simulink model "My_System"  (R2022b)
settings: Solver=ode4  StartTime=0.0  StopTime=10.0  FixedStep=0.01  RelTol=1e-3  EnableMultiTasking=on
Description:
  | Real-Time Van der Pol Simulation
  | 
  | This demonstration shows a real-time version of the Simulink Van der Pol
  | simulation demo. This model does not need any external signals, so it does
  | not need any data acquisition hardware or driver. This makes the model ideal
  | for first experiments with Real-Time Windows Target, without need to
  | worry about proper I/O hardware configuration.
  | 
  | How to run this demo:
  | 
  |   1. Build the model using Tools -> Real-Time Workshop -> Build Model.
  |   2. Connect to the real-time code using Simulation -> Connect to target.
  |   3. Start the real-time execution using Simulation -> Start real-time code.
settings Model: SimulationMode=external  Creator=Houska  LastModifiedBy=artur
settings SolverCC: AlgebraicLoopSolver=TrustRegion
settings DataIOCC: LimitDataPoints=on  SaveFormat=Array  SignalLoggingSaveFormat=ModelDataLogs  SaveOutput=off  SaveTime=off  ReturnWorkspaceOutputs=off  SignalLoggingName=logsOut
settings OptimizationCC: ExpressionDepthLimit=2147483647  InitFltsAndDblsToZero=on
settings DebuggingCC: SaveWithParameterizedLinksMsg=none  UnderspecifiedInitializationDetection=Classic  MergeDetectMultiDrivingBlocksExec=none  SignalResolutionControl=TryResolveAllWithWarning  MultiTaskDSMMsg=warning  MultiTaskCondExecSysMsg=none  FcnCallInpInsideContextMsg=warning  UnconnectedInputMsg=warning  UnconnectedOutputMsg=warning  UnconnectedLineMsg=warning  AllowSymbolicDim=off  StateNameClashWarn=warning  PregeneratedLibrarySubsystemCodeDiagnostic=none  SFUnexpectedBacktrackingDiag=warning  SFNoUnconditionalDefaultTransitionDiag=warning  SFExecutionAtInitializationDiag=none  SFMachineParentedDataDiag=warning  ArithmeticOperatorsInVariantConditions=warning
settings HardwareCC: ProdBitPerPointer=32  ProdBitPerSizeT=32  ProdBitPerPtrDiffT=32  ProdLargestAtomicFloat=None  ProdWordSize=32  ProdHWDeviceType=32-bit Real-Time Windows Target  TargetHWDeviceType=32-bit Generic  ProdEqTarget=off
settings ModelReferenceCC: EnableRefExpFcnMdlSchedulingChecks=on  PropagateSignalLabelsOutOfModel=off
settings SFSimCC: SimUseLocalCustomCode=off  CustomCodeUndefinedFunction=UseInterfaceOnly
settings RTWCC: Description=servo (Visual C/C++)  SystemTargetFile=rtcon_servo_usb2.tlc  TemplateMakefile=servo_vc_usb2_x64.tmf  RTWUseLocalCustomCode=off  DLArmComputeVersion=19.05
settings CodeAppCC: StateflowObjectComments=on
settings STFCustomTargetCC: ModelReferenceCompliant=off  CombineOutputUpdateFcns=on  MatFileLogging=on  SystemTargetFile=rtcon_servo_usb2.tlc
settings GRTTargetCC: TargetLangStandard=C89/C90 (ANSI)  ModelReferenceCompliant=off  ParMdlRefBuildCompliant=off  CompOptLevelCompliant=off  ConcurrentExecutionCompliant=off  CPPClassGenCompliant=off  UseToolchainInfoCompliant=off  ExtMode=on  ExtModeMexFile=rtcon_ext_comm
settings ConfigComp: CovMetricSettings=dw  CovSaveCumulativeToWorkspaceVar=on  CovSaveSingleToWorkspaceVar=on  CovExternalEMLEnable=off  CovSFcnEnable=off

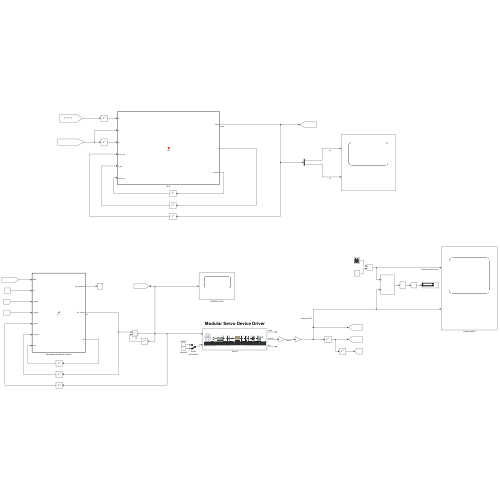
[thumbnail: Simulink's stored preview of the top-level diagram]
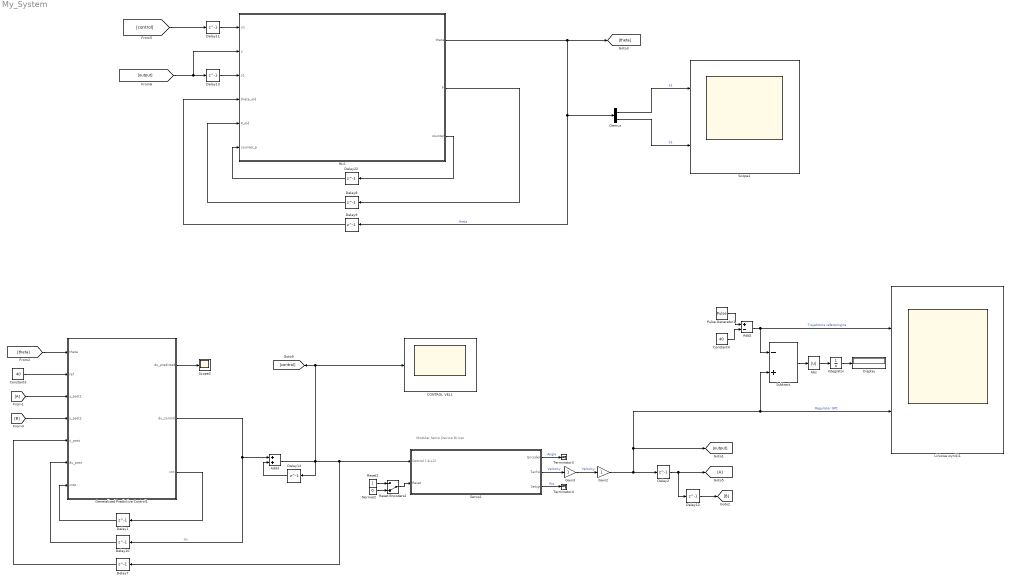
== system My_System ==
  note: Modular Servo Device Driver
  Abs : Abs  SaturateOnIntegerOverflow=off
  Add2 : Sum  Inputs=+-
  Add3 : Sum
  CONTROL VEL1 : Scope
  Constant3 : Constant  Value=40
  Constant4 : Constant  Value=40
  Delay1 : Delay  DelayLength=1  InitialCondition=1
  Delay{2,7,10..14} (7 alike) : Delay  DelayLength=1  InitialCondition=0
  Delay22 : Delay  DelayLength=1  InitialCondition=10
  Delay8 : Delay  DelayLength=1  InitialCondition=eye(2) * 10^6
  Delay9 : Delay  DelayLength=1  InitialCondition=[0.79 1.9048]
  Demux : Demux  Outputs=2
  Display : Display
  From1 : From
  Gain2 : Gain
  Gain3 : Gain
  Generalized Predictive Control1 : MATLAB Function  TreatAsAtomicUnit=on
  Goto5 : Goto
  Integrator : Integrator
  Liniowe wyniki1 : Scope  NumInputPorts=2
  Normal2 : Constant  Value=0
  Pulse Generator1 : DiscretePulseGenerator  PulseType=Time based  Amplitude=80  Period=4  PulseWidth=50
  RLS : MATLAB Function  TreatAsAtomicUnit=on
  Reset Encoders2 : ManualSwitch  CurrentSetting=0
  Reset2 : Constant
  Scope1 : Scope  NumInputPorts=2
  Scope2 : Scope
  Servo2 : Subsystem
      mask Display: image(imread('Servo_inteco.JPG'))
  Subtract : Sum  Inputs=-+
  Terminator3 : Terminator
  Terminator4 : Terminator
  wires:
  [control] -> Delay11/1
  RLS/1(theta) -> Demux/1, Delay9/1, [theta]  "theta"
  Delay9/1 -> RLS/4(theta_old)
  Delay8/1 -> RLS/5(P_old)
  [output] -> Delay13/1, RLS/2(y)
  Demux/2 -> Scope1/2  "b1"
  Delay13/1 -> RLS/3(y1)
  Delay22/1 -> RLS/6(counter_p)
  RLS/3(counter) -> Delay22/1
  Delay11/1 -> RLS/1(u1)
  Demux/1 -> Scope1/1  "a1"
  RLS/2(P) -> Delay8/1
  Generalized Predictive Control1/1(du_predicted) -> Scope2/1
  [B] -> Generalized Predictive Control1/4(y_past2)
  From1/1 -> Generalized Predictive Control1/3(y_past1)
  Generalized Predictive Control1/3(cnt) -> Delay1/1
  Gain2/1 -> Delay2/1, [output], Liniowe wyniki1/2, Subtract/2  "Regulator GPC"
  Constant4/1 -> Add2/2
  Delay12/1 -> [B]
  Delay2/1 -> Delay12/1, Goto5/1
  Subtract/1 -> Abs/1
  Delay10/1 -> Generalized Predictive Control1/6(du_past)
  Delay14/1 -> Add3/2
  [theta] -> Generalized Predictive Control1/1(theta)
  Generalized Predictive Control1/2(du_control) -> Delay10/1, Add3/1  "du"
  Add2/1 -> Liniowe wyniki1/1, Subtract/1  "Trajektoria referencyjna"
  Delay7/1 -> Generalized Predictive Control1/5(u_past)
  Delay1/1 -> Generalized Predictive Control1/7(cntp)
  Abs/1 -> Integrator/1
  Constant3/1 -> Generalized Predictive Control1/2(ref)
  Gain3/1 -> Gain2/1  "Velocity"
  Pulse Generator1/1 -> Add2/1
  Integrator/1 -> Display/1
  Servo2/2(Tacho) -> Gain3/1  "Velocity"
  Servo2/3(Setup) -> Terminator4/1  "Pot"
  Add3/1 -> [control], CONTROL VEL1/1, Servo2/1(Control (-1/+1)), Delay7/1, Delay14/1
  Reset Encoders2/1 -> Servo2/2(Reset)
  Servo2/1(Encoder) -> Terminator3/1  "Angle"
  Normal2/1 -> Reset Encoders2/2
  Reset2/1 -> Reset Encoders2/1

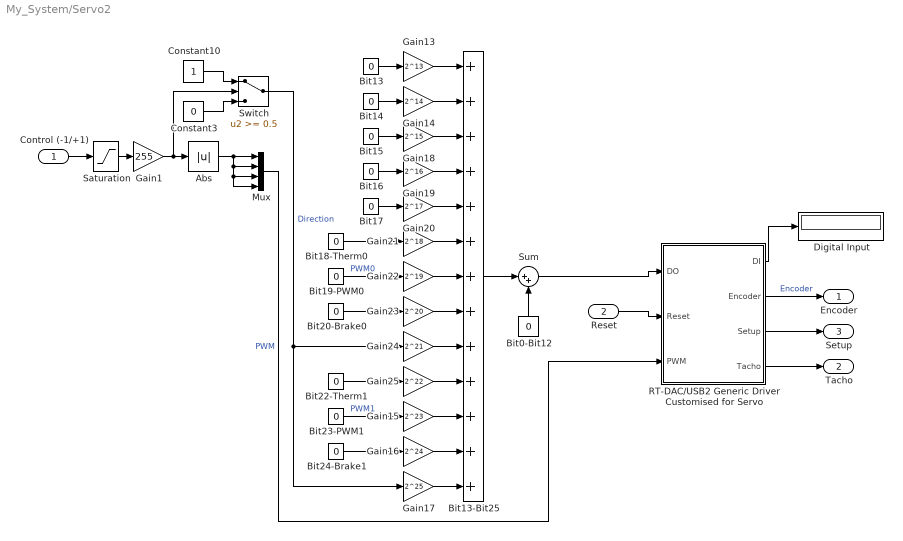
== system My_System/Servo2 ==
  Control (-1/+1) : Inport
  Reset : Inport  Port=2
  Abs : Abs
  Bit0-Bit12 : Constant  Value=0
  Bit{13..17} (5 alike) : Constant  Value=0
  Bit13-Bit25 : Sum  Inputs=+++++++++++++  InputSameDT=on  SaturateOnIntegerOverflow=on  OutDataTypeStr=Inherit: Same as first input
  Bit18-Therm0 : Constant  Value=0
  Bit19-PWM0 : Constant  Value=0
  Bit20-Brake0 : Constant  Value=0
  Bit22-Therm1 : Constant  Value=0
  Bit23-PWM1 : Constant  Value=0
  Bit24-Brake1 : Constant  Value=0
  Constant10 : Constant
  Constant3 : Constant  Value=0
  Digital Input : Display
  Gain1 : Gain  Gain=255  SaturateOnIntegerOverflow=on  OutDataTypeStr=Inherit: Same as input  ParamDataTypeStr=Inherit: Same as input
  Gain13 : Gain  Gain=2^13  SaturateOnIntegerOverflow=on  OutDataTypeStr=Inherit: Same as input  ParamDataTypeStr=Inherit: Same as input
  Gain14 : Gain  Gain=2^14  SaturateOnIntegerOverflow=on  OutDataTypeStr=Inherit: Same as input  ParamDataTypeStr=Inherit: Same as input
  Gain15 : Gain  Gain=2^23  SaturateOnIntegerOverflow=on  OutDataTypeStr=Inherit: Same as input  ParamDataTypeStr=Inherit: Same as input
  Gain16 : Gain  Gain=2^24  SaturateOnIntegerOverflow=on  OutDataTypeStr=Inherit: Same as input  ParamDataTypeStr=Inherit: Same as input
  Gain17 : Gain  Gain=2^25  SaturateOnIntegerOverflow=on  OutDataTypeStr=Inherit: Same as input  ParamDataTypeStr=Inherit: Same as input
  Gain18 : Gain  Gain=2^15  SaturateOnIntegerOverflow=on  OutDataTypeStr=Inherit: Same as input  ParamDataTypeStr=Inherit: Same as input
  Gain19 : Gain  Gain=2^16  SaturateOnIntegerOverflow=on  OutDataTypeStr=Inherit: Same as input  ParamDataTypeStr=Inherit: Same as input
  Gain20 : Gain  Gain=2^17  SaturateOnIntegerOverflow=on  OutDataTypeStr=Inherit: Same as input  ParamDataTypeStr=Inherit: Same as input
  Gain21 : Gain  Gain=2^18  SaturateOnIntegerOverflow=on  OutDataTypeStr=Inherit: Same as input  ParamDataTypeStr=Inherit: Same as input
  Gain22 : Gain  Gain=2^19  SaturateOnIntegerOverflow=on  OutDataTypeStr=Inherit: Same as input  ParamDataTypeStr=Inherit: Same as input
  Gain23 : Gain  Gain=2^20  SaturateOnIntegerOverflow=on  OutDataTypeStr=Inherit: Same as input  ParamDataTypeStr=Inherit: Same as input
  Gain24 : Gain  Gain=2^21  SaturateOnIntegerOverflow=on  OutDataTypeStr=Inherit: Same as input  ParamDataTypeStr=Inherit: Same as input
  Gain25 : Gain  Gain=2^22  SaturateOnIntegerOverflow=on  OutDataTypeStr=Inherit: Same as input  ParamDataTypeStr=Inherit: Same as input
  Mux : Mux
  RT-DAC/USB2 Generic Driver Customised for Servo : Subsystem
      mask Display: disp('RT-DAC/USB2\n\nGeneric Driver\nVersion 2.1')
  Saturation : Saturate  UpperLimit=1  LowerLimit=-1
  Sum : Sum  Inputs=|++  InputSameDT=on  SaturateOnIntegerOverflow=on  OutDataTypeStr=Inherit: Same as first input
  Switch : Switch  Threshold=0.5  SaturateOnIntegerOverflow=off
  Encoder : Outport  VectorParamsAs1DForOutWhenUnconnected=off
  Tacho : Outport  Port=2  VectorParamsAs1DForOutWhenUnconnected=off
  Setup : Outport  Port=3  VectorParamsAs1DForOutWhenUnconnected=off
  wires:
  RT-DAC/USB2 Generic Driver Customised for Servo/4(Tacho) -> Tacho/1
  RT-DAC/USB2 Generic Driver Customised for Servo/3(Setup) -> Setup/1
  RT-DAC/USB2 Generic Driver Customised for Servo/2(Encoder) -> Encoder/1  "Encoder"
  Mux/1 -> RT-DAC/USB2 Generic Driver Customised for Servo/3(PWM)  "PWM"
  Switch/1 -> Gain17/1, Gain24/1  "Direction"
  Abs/1 -> Mux/4, Mux/3, Mux/2, Mux/1
  Constant3/1 -> Switch/3
  Constant10/1 -> Switch/1
  Gain1/1 -> Switch/2, Abs/1
  Saturation/1 -> Gain1/1
  Control (-1/+1)/1 -> Saturation/1
  Reset/1 -> RT-DAC/USB2 Generic Driver Customised for Servo/2(Reset)
  Bit24-Brake1/1 -> Gain16/1
  Bit23-PWM1/1 -> Gain15/1  "PWM1"
  Bit22-Therm1/1 -> Gain25/1
  Bit13-Bit25/1 -> Sum/1
  Sum/1 -> RT-DAC/USB2 Generic Driver Customised for Servo/1(DO)
  Gain17/1 -> Bit13-Bit25/13
  Gain16/1 -> Bit13-Bit25/12
  Gain15/1 -> Bit13-Bit25/11
  Gain25/1 -> Bit13-Bit25/10
  Gain24/1 -> Bit13-Bit25/9
  Gain23/1 -> Bit13-Bit25/8
  Gain22/1 -> Bit13-Bit25/7
  Gain21/1 -> Bit13-Bit25/6
  Gain20/1 -> Bit13-Bit25/5
  Gain19/1 -> Bit13-Bit25/4
  Gain18/1 -> Bit13-Bit25/3
  Gain14/1 -> Bit13-Bit25/2
  Gain13/1 -> Bit13-Bit25/1
  Bit0-Bit12/1 -> Sum/2
  RT-DAC/USB2 Generic Driver Customised for Servo/1(DI) -> Digital Input/1
  Bit20-Brake0/1 -> Gain23/1
  Bit19-PWM0/1 -> Gain22/1  "PWM0"
  Bit18-Therm0/1 -> Gain21/1
  Bit17/1 -> Gain20/1
  Bit16/1 -> Gain19/1
  Bit15/1 -> Gain18/1
  Bit14/1 -> Gain14/1
  Bit13/1 -> Gain13/1

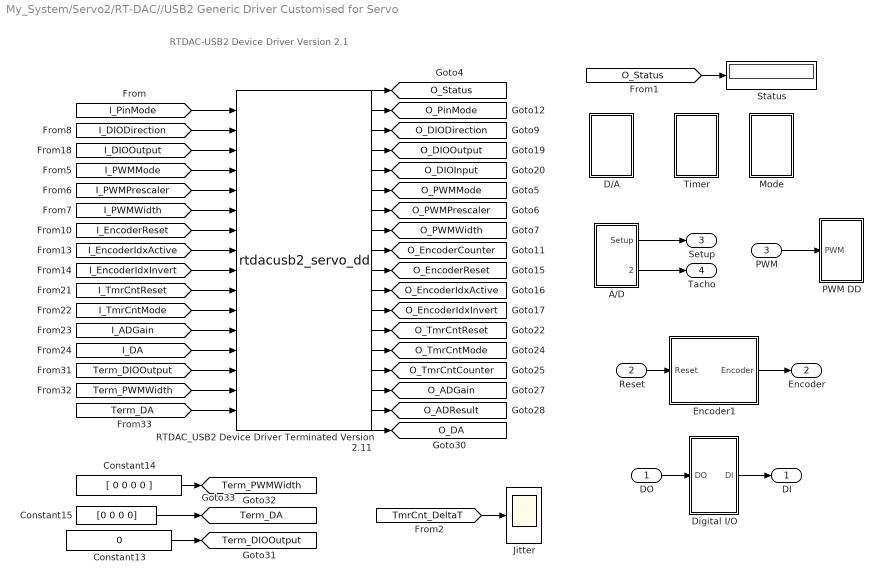
== system My_System/Servo2/RT-DAC//USB2 Generic Driver Customised for Servo ==
  note: RTDAC-USB2 Device Driver
      | Version 2.1
  DO : Inport
  Reset : Inport  Port=2
  PWM : Inport  Port=3
  A/D : Subsystem
  Constant13 : Constant  Value=0
  Constant14 : Constant  Value=[ 0 0 0 0 ]
  Constant15 : Constant  Value=[0 0 0 0]
  D/A : Subsystem
  Digital I/O : Subsystem
  Encoder1 : Subsystem
  Jitter : Scope
  Mode : Subsystem
  PWM DD : Subsystem
  RTDAC_USB2 Device Driver Terminated Version 2.11 : S-Function  FunctionName=rtdacusb2_servo_dd  Parameters=0.01  SFunctionDeploymentMode=off  EnableBusSupport=off
  Status : Display
  Timer : Subsystem
  DI : Outport  VectorParamsAs1DForOutWhenUnconnected=off
  Encoder : Outport  Port=2  VectorParamsAs1DForOutWhenUnconnected=off
  Setup : Outport  Port=3  VectorParamsAs1DForOutWhenUnconnected=off
  Tacho : Outport  Port=4  VectorParamsAs1DForOutWhenUnconnected=off
  tag scope: O_ADGain=global, O_ADResult=global, O_DA=global, O_DIODirection=global, O_DIOInput=global, O_DIOOutput=global, O_EncoderCounter=global, O_EncoderIdxActive=global, O_EncoderIdxInvert=global, O_EncoderReset=global, O_PWMMode=global, O_PWMPrescaler=global, O_PWMWidth=global, O_PinMode=global, O_Status=global, O_TmrCntCounter=global, O_TmrCntMode=global, O_TmrCntReset=global, Term_DA=global, Term_DIOOutput=global, Term_PWMWidth=global
  wires:
  [TmrCnt_DeltaT] -> Jitter/1
  Constant14/1 -> [Term_PWMWidth]
  [Term_DA] -> RTDAC_USB2 Device Driver Terminated Version 2.11/16
  [Term_PWMWidth] -> RTDAC_USB2 Device Driver Terminated Version 2.11/15
  [Term_DIOOutput] -> RTDAC_USB2 Device Driver Terminated Version 2.11/14
  Constant13/1 -> [Term_DIOOutput]
  Constant15/1 -> [Term_DA]
  A/D/2(Tacho) -> Tacho/1
  A/D/1(Setup) -> Setup/1
  Reset/1 -> Encoder1/1(Reset)
  Digital I/O/1(DI) -> DI/1
  DO/1 -> Digital I/O/1(DO)
  Encoder1/1(Encoder) -> Encoder/1
  RTDAC_USB2 Device Driver Terminated Version 2.11/5 -> [O_DIOInput]
  RTDAC_USB2 Device Driver Terminated Version 2.11/4 -> [O_DIOOutput]
  [I_DIOOutput] -> RTDAC_USB2 Device Driver Terminated Version 2.11/3
  RTDAC_USB2 Device Driver Terminated Version 2.11/12 -> [O_EncoderIdxInvert]
  RTDAC_USB2 Device Driver Terminated Version 2.11/11 -> [O_EncoderIdxActive]
  RTDAC_USB2 Device Driver Terminated Version 2.11/10 -> [O_EncoderReset]
  [I_EncoderIdxInvert] -> RTDAC_USB2 Device Driver Terminated Version 2.11/9
  [I_EncoderIdxActive] -> RTDAC_USB2 Device Driver Terminated Version 2.11/8
  RTDAC_USB2 Device Driver Terminated Version 2.11/2 -> [O_PinMode]
  RTDAC_USB2 Device Driver Terminated Version 2.11/3 -> [O_DIODirection]
  RTDAC_USB2 Device Driver Terminated Version 2.11/9 -> [O_EncoderCounter]
  [I_EncoderReset] -> RTDAC_USB2 Device Driver Terminated Version 2.11/7
  [I_DIODirection] -> RTDAC_USB2 Device Driver Terminated Version 2.11/2
  [I_PWMWidth] -> RTDAC_USB2 Device Driver Terminated Version 2.11/6
  [I_PWMPrescaler] -> RTDAC_USB2 Device Driver Terminated Version 2.11/5
  [I_PWMMode] -> RTDAC_USB2 Device Driver Terminated Version 2.11/4
  RTDAC_USB2 Device Driver Terminated Version 2.11/8 -> [O_PWMWidth]
  RTDAC_USB2 Device Driver Terminated Version 2.11/7 -> [O_PWMPrescaler]
  RTDAC_USB2 Device Driver Terminated Version 2.11/6 -> [O_PWMMode]
  [O_Status] -> Status/1
  RTDAC_USB2 Device Driver Terminated Version 2.11/1 -> [O_Status]
  PWM/1 -> PWM DD/1(PWM)
  [I_PinMode] -> RTDAC_USB2 Device Driver Terminated Version 2.11/1
  [I_TmrCntReset] -> RTDAC_USB2 Device Driver Terminated Version 2.11/10
  [I_ADGain] -> RTDAC_USB2 Device Driver Terminated Version 2.11/12
  [I_TmrCntMode] -> RTDAC_USB2 Device Driver Terminated Version 2.11/11
  [I_DA] -> RTDAC_USB2 Device Driver Terminated Version 2.11/13
  RTDAC_USB2 Device Driver Terminated Version 2.11/13 -> [O_TmrCntReset]
  RTDAC_USB2 Device Driver Terminated Version 2.11/14 -> [O_TmrCntMode]
  RTDAC_USB2 Device Driver Terminated Version 2.11/15 -> [O_TmrCntCounter]
  RTDAC_USB2 Device Driver Terminated Version 2.11/16 -> [O_ADGain]
  RTDAC_USB2 Device Driver Terminated Version 2.11/17 -> [O_ADResult]
  RTDAC_USB2 Device Driver Terminated Version 2.11/18 -> [O_DA]

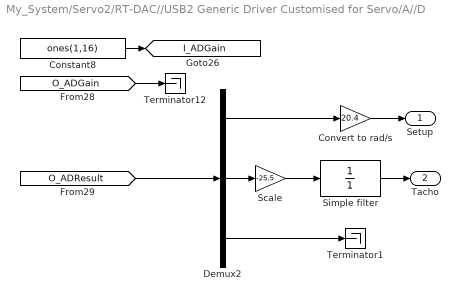
== system My_System/Servo2/RT-DAC//USB2 Generic Driver Customised for Servo/A//D ==
  Constant8 : Constant  Value=ones(1,16)
  Convert to rad/s : Gain  Gain=20.4  OutDataTypeStr=Inherit: Same as input  ParamDataTypeStr=Inherit: Same as input
  Demux2 : Demux  Outputs=[1 1 14]
      settings: DisplayOption=none
  Scale : Gain  Gain=-25.5  OutDataTypeStr=Inherit: Same as input  ParamDataTypeStr=Inherit: Same as input
  Simple filter : TransferFcn  Denominator=[0.0 1]
  Terminator1 : Terminator
  Terminator12 : Terminator
  Setup : Outport  InitialOutput=0  VectorParamsAs1DForOutWhenUnconnected=off
  Tacho : Outport  Port=2  InitialOutput=0  VectorParamsAs1DForOutWhenUnconnected=off
  tag scope: I_ADGain=global
  wires:
  Scale/1 -> Simple filter/1
  Demux2/3 -> Terminator1/1
  Simple filter/1 -> Tacho/1
  Convert to rad/s/1 -> Setup/1
  Demux2/1 -> Convert to rad/s/1
  Demux2/2 -> Scale/1
  Constant8/1 -> [I_ADGain]
  [O_ADGain] -> Terminator12/1
  [O_ADResult] -> Demux2/1

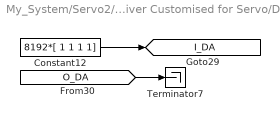
== system My_System/Servo2/RT-DAC//USB2 Generic Driver Customised for Servo/D//A ==
  Constant12 : Constant  Value=8192*[ 1 1 1 1]
  Terminator7 : Terminator
  tag scope: I_DA=global
  wires:
  [O_DA] -> Terminator7/1
  Constant12/1 -> [I_DA]

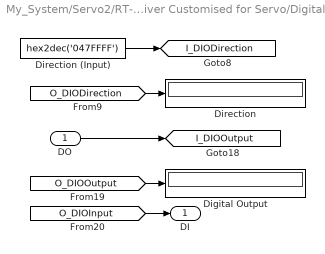
== system My_System/Servo2/RT-DAC//USB2 Generic Driver Customised for Servo/Digital I//O ==
  DO : Inport
  Digital Output : Display
  Direction : Display
  Direction (Input) : Constant  Value=hex2dec('047FFFF')
  DI : Outport  VectorParamsAs1DForOutWhenUnconnected=off
  tag scope: I_DIODirection=global, I_DIOOutput=global
  wires:
  [O_DIOInput] -> DI/1
  [O_DIOOutput] -> Digital Output/1
  DO/1 -> [I_DIOOutput]
  [O_DIODirection] -> Direction/1
  Direction (Input)/1 -> [I_DIODirection]

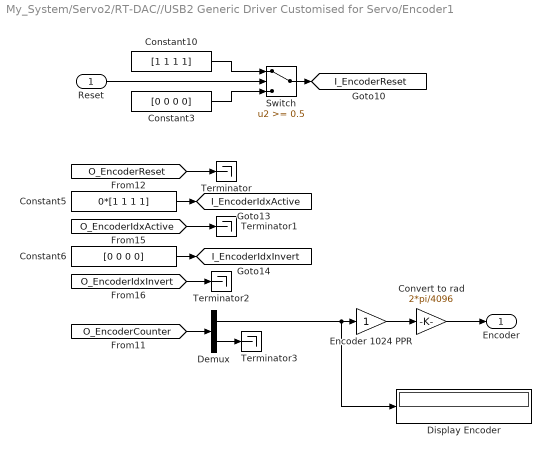
== system My_System/Servo2/RT-DAC//USB2 Generic Driver Customised for Servo/Encoder1 ==
  Reset : Inport
  Constant10 : Constant  Value=[1 1 1 1]
  Constant3 : Constant  Value=[0 0 0 0]
  Constant5 : Constant  Value=0*[1 1 1 1]
  Constant6 : Constant  Value=[0 0 0 0]
  Convert to rad : Gain  Gain=2*pi/4096  SaturateOnIntegerOverflow=on  OutDataTypeStr=Inherit: Same as input  ParamDataTypeStr=Inherit: Same as input
  Demux : Demux  Outputs=[1 3]
  Display Encoder : Display
  Encoder 1024 PPR : Gain  SaturateOnIntegerOverflow=on  OutDataTypeStr=Inherit: Same as input  ParamDataTypeStr=Inherit: Same as input
  Switch : Switch  Threshold=0.5  SaturateOnIntegerOverflow=off
  Terminator{,1..3} (4 alike) : Terminator
  Encoder : Outport  VectorParamsAs1DForOutWhenUnconnected=off
  tag scope: I_EncoderIdxActive=global, I_EncoderIdxInvert=global, I_EncoderReset=global
  wires:
  Convert to rad/1 -> Encoder/1
  Demux/1 -> Encoder 1024 PPR/1, Display Encoder/1
  Encoder 1024 PPR/1 -> Convert to rad/1
  Reset/1 -> Switch/2
  Constant3/1 -> Switch/3
  Constant10/1 -> Switch/1
  Switch/1 -> [I_EncoderReset]
  Demux/2 -> Terminator3/1
  [O_EncoderIdxInvert] -> Terminator2/1
  [O_EncoderIdxActive] -> Terminator1/1
  Constant6/1 -> [I_EncoderIdxInvert]
  Constant5/1 -> [I_EncoderIdxActive]
  [O_EncoderReset] -> Terminator/1
  [O_EncoderCounter] -> Demux/1

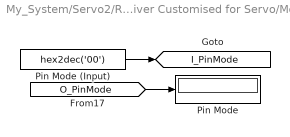
== system My_System/Servo2/RT-DAC//USB2 Generic Driver Customised for Servo/Mode ==
  Pin Mode : Display
  Pin Mode (Input) : Constant  Value=hex2dec('00')
  tag scope: I_PinMode=global
  wires:
  Pin Mode (Input)/1 -> [I_PinMode]
  [O_PinMode] -> Pin Mode/1

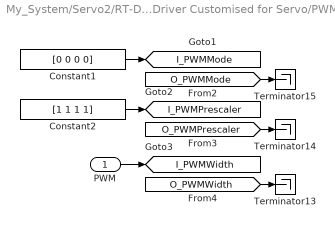
== system My_System/Servo2/RT-DAC//USB2 Generic Driver Customised for Servo/PWM DD ==
  PWM : Inport
  Constant1 : Constant  Value=[0 0 0 0]
  Constant2 : Constant  Value=[1 1 1 1]
  Terminator13 : Terminator
  Terminator14 : Terminator
  Terminator15 : Terminator
  tag scope: I_PWMMode=global, I_PWMPrescaler=global, I_PWMWidth=global
  wires:
  PWM/1 -> [I_PWMWidth]
  [O_PWMWidth] -> Terminator13/1
  [O_PWMPrescaler] -> Terminator14/1
  [O_PWMMode] -> Terminator15/1
  Constant2/1 -> [I_PWMPrescaler]
  Constant1/1 -> [I_PWMMode]

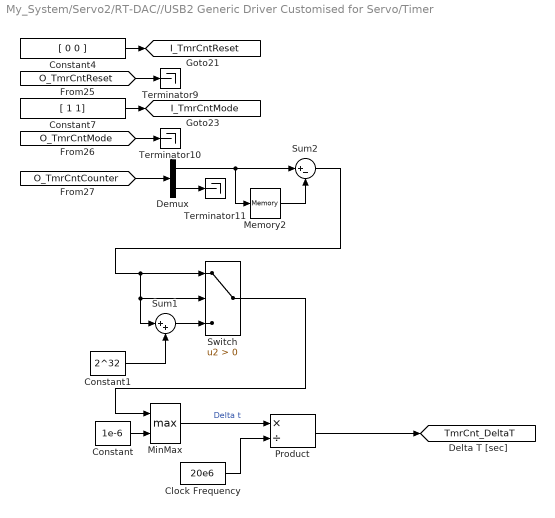
== system My_System/Servo2/RT-DAC//USB2 Generic Driver Customised for Servo/Timer ==
  Clock Frequency : Constant  Value=20e6
  Constant : Constant  Value=1e-6
  Constant1 : Constant  Value=2^32
  Constant4 : Constant  Value=[ 0 0 ]
  Constant7 : Constant  Value=[ 1 1]
  Demux : Demux  Outputs=2
      settings: DisplayOption=none
  Memory2 : Memory
  MinMax : MinMax  Function=max  Inputs=2  InputSameDT=on  SaturateOnIntegerOverflow=on
  Product : Product  Inputs=*/  SaturateOnIntegerOverflow=on  OutDataTypeStr=Inherit: Same as first input
  Sum1 : Sum  Inputs=|++  InputSameDT=on  SaturateOnIntegerOverflow=on  OutDataTypeStr=Inherit: Same as first input
  Sum2 : Sum  Inputs=|+-  InputSameDT=on  SaturateOnIntegerOverflow=on  OutDataTypeStr=Inherit: Same as first input
  Switch : Switch  Criteria=u2 > Threshold
  Terminator10 : Terminator
  Terminator11 : Terminator
  Terminator9 : Terminator
  tag scope: I_TmrCntMode=global, I_TmrCntReset=global, TmrCnt_DeltaT=global
  wires:
  Demux/2 -> Terminator11/1
  Demux/1 -> Sum2/1, Memory2/1
  Switch/1 -> MinMax/1
  Constant1/1 -> Sum1/2
  Sum1/1 -> Switch/3
  Sum2/1 -> Sum1/1, Switch/2, Switch/1
  Clock Frequency/1 -> Product/2
  MinMax/1 -> Product/1  "Delta t"
  Product/1 -> [TmrCnt_DeltaT]
  [O_TmrCntCounter] -> Demux/1
  Memory2/1 -> Sum2/2
  Constant/1 -> MinMax/2
  Constant4/1 -> [I_TmrCntReset]
  [O_TmrCntReset] -> Terminator9/1
  Constant7/1 -> [I_TmrCntMode]
  [O_TmrCntMode] -> Terminator10/1

== matlab function My_System/Generalized Predictive Control1 ==
  data: du_predicted output; theta input; ref input; y_past1 input; y_past2 input; u_past input; du_past input; du_control output; cntp input; cnt output
function [du_predicted, du_control,cnt] = fcn(theta,ref,y_past1,y_past2,u_past,du_past,cntp)

cnt = cntp;

%Współczynniki modelu z algorytmu RLS
a1 = -theta(1);
b1 = theta(2);

%Przeszłe wyjścia
y_past = [y_past1;y_past2];
    
%Parametry
ny = 32; %HORYZONT PREDYKCJI
nu = 12; %HORYZONT STEROWANIA
lambda = 0.5;
    
%Czy wykorzystać T-filtr?
filtrowanie = false;
    
%Ustawienie ograniczeń dla optymalizatora 
%true - ograniczenia na y, false - bez ograniczeń na y
ograniczenie_wyjscia = true;

du_max = 1;
du_min = -1;
u_max = 1;
u_min = -1;
y_max = 42;
y_min = -42;

%Trajektoria referencyjna, stała
Ts = 0.01; %PRÓBKOWANIE SYMULACJI
sim_time = 4; %CZAS SYMULACJI

traj_ub = ref*ones(1/Ts*sim_time/2,1);

traj_lb = -ref*ones(1/Ts*sim_time/2,1);

trajektoria = [traj_ub;traj_lb;traj_ub;-ref*ones(ny,1)];

ref = trajektoria(cnt:ny+cnt-1, 1);

cnt = cntp + 1;

%%%



    %Wyznaczenie wielomianów a i b
    a = [1 a1];
    b = [0 b1];
    A = conv(a,[1 -1]);
    
    %Wyznaczenie macierzy predykcji
    [Ca,Ha] = predmat(A,ny);
    [Cb,Hb] = predmat(b,ny);
    
    Cai = inv(Ca);
    
    H = Cai*Cb;
    P = Cai*Hb;
    Q = Cai*(-Ha);

%%%%%%%%%%%%%%%%%%%%%%%%%%%%%%%%%%%%%%%%%%%%%%%%%%%%%%%%%%%%%%%%%%%%%%%%%%%

if filtrowanie == true
    Tfilt = [1 -0.2];
    
    [Ct,Ht] = predmat(Tfilt,ny);
    Pfilt = Ct * P - H * Ht;
    Qfilt = Ct * Q + Ht;
    
    P = Pfilt;
    Q = Qfilt;
end

%%%%%%%%%%%%%%%%%%%%%%%%%%%%%%%%%%%%%%%%%%%%%%%%%%%%%%%%%%%%%%%%%%%%%%%%%%%

    Hu = H(:,1:nu); %horyzont sterowania

%Prawo sterowania dla algorytmu z ograniczeniami
    S = Hu'*Hu + eye(nu)*lambda;
    S = (S + S')/2;
    f = Hu'*Q * y_past + Hu'*P * du_past - Hu' * ref;

    if ograniczenie_wyjscia == true
        %OGRANICZENIA Z Y
        [C,dd,du,ddu,dy] = mpc_ograniczenia(du_max, du_min,u_max,u_min,y_max,y_min,nu,Hu,P,Q,1,2);
        dt = dd + du * u_past + ddu * du_past + dy*y_past;
    else
        %OGRANICZENIA BEZ Y
        [C, dd,du] = mpc_ograniczenia_bez_y(du_max,du_min,u_max,u_min,nu);
        dt = dd + du * u_past;
    end


    opts = optimoptions('quadprog','Algorithm','active-set');

    x0 = 0.1*eye(nu,1);

    du_predicted = quadprog(S,f,C,dt,[],[],[],[],x0,opts);

    du_control = du_predicted(1);


%Prawo sterowania dla algorytmu bez ograniczeń
% Pr = ( inv(Hu'*Hu+lambda*eye(nu)) ) * Hu';
% Nk = Pr*Q;
% Dk = Pr*P;
% 
% du_predicted = Pr * ref - Dk * du_past - Nk*y_past;
% du_control = du_predicted(1);

== matlab function My_System/RLS ==
  data: u1 input; y input; y1 input; theta output; theta_old input; P_old input; P output; counter_p input; counter output
function [theta,P,counter]= fcn(u1,y,y1,theta_old,P_old,counter_p)

counter = counter_p;

if counter_p == 10

lambda = 0.985;
phi = [y1;u1];

K = P_old * phi/(lambda + phi'*P_old*phi);

P = ((eye(2) - K * phi') * P_old) * lambda^-1;

theta = theta_old + K * (y - phi'*theta_old);

counter = 0;
else
    theta = theta_old;
    P = P_old;
    counter = counter + 1;
end
